simulink model "generic_IVS"  (R2024a)
settings: Solver=FixedStepDiscrete  StartTime=0.0  StopTime=inf  FixedStep=0.001  RelTol=1e-3  EnableMultiTasking=on
model workspace (MAT data in the model file):
  APPROACH = [-49.2532697283 -46.8560638421 -44.4231792578 -41.9812023919 -38.6885385845 -35.362557161 -32.0241539117 -28.6853351363 -25.3485360015 -22.0129625698 -18.6780310991 -15.3435011563 ... (76 elements, 38x2)]
  LANE_LEN = [284; 276; 267]
  LANE_XY = [59.0003214677 62.3317238784 65.6577746803 68.9711287644 72.2614514234 75.5172879138 77.9296982442 80.3117765819 82.6592727002 84.9682672017 87.2351542049 89.4565910317 ... (1704 elements, 284x2x3)]
  N_LANE = 3
  PARK_OCC = [1 1 1 1 1 1 1 1 1 1 1 1 ... (40000 elements, 200x200)]
  WB = 2.9
  branch_lane = 3
  branch_x = -49.2532697283
  branch_y = 17.3349288561
  cruise_lane = 1
  entrance_x = 6
  entrance_y = -36.6
  lane_width = 3.5
  park_goal = [21.4; -44.3; 1.57079632679]
  toll_lane = 1
  toll_post = 20
  toll_pre = 45
  toll_station = 202.6
  toll_x = -176.17
  toll_y = -85.66
  v_cruise = 11
  v_park = 2.78
  waypoints = [-81.8048181182 -79.1416974235 -76.4199514846 -73.3097017696 -70.5703457405 -67.625901331 -64.4903894371 -61.1945301864 -57.8351626085 -54.4642235015 -51.0966947204 -47.7361432477 ... (1754 elements, 877x2)]
libraries: CarMaker4SL x57, simulink x1
(part 4 of 4)

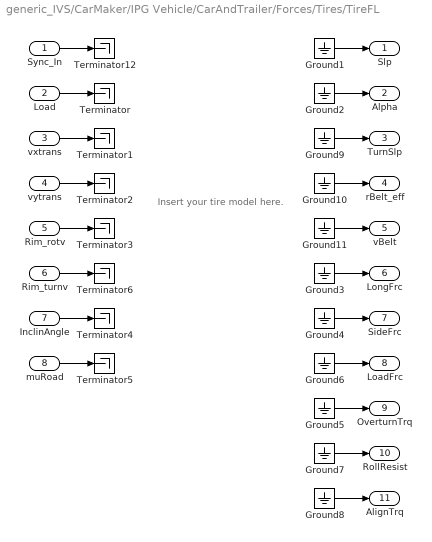
== system generic_IVS/CarMaker/IPG Vehicle/CarAndTrailer/Forces/Tires/TireFL ==
  note: Insert your tire model here.
  Sync_In : Inport
  Load : Inport  Port=2
  vxtrans : Inport  Port=3
  vytrans : Inport  Port=4
  Rim_rotv : Inport  Port=5
  Rim_turnv : Inport  Port=6
  InclinAngle : Inport  Port=7
  muRoad : Inport  Port=8
  Ground{1..11} (11 alike) : Ground
  Terminator{,1..6,12} (8 alike) : Terminator
  Slp : Outport  VectorParamsAs1DForOutWhenUnconnected=off
  Alpha : Outport  Port=2  VectorParamsAs1DForOutWhenUnconnected=off
  TurnSlp : Outport  Port=3  VectorParamsAs1DForOutWhenUnconnected=off
  rBelt_eff : Outport  Port=4  VectorParamsAs1DForOutWhenUnconnected=off
  vBelt : Outport  Port=5  VectorParamsAs1DForOutWhenUnconnected=off
  LongFrc : Outport  Port=6  VectorParamsAs1DForOutWhenUnconnected=off
  SideFrc : Outport  Port=7  VectorParamsAs1DForOutWhenUnconnected=off
  LoadFrc : Outport  Port=8  VectorParamsAs1DForOutWhenUnconnected=off
  OverturnTrq : Outport  Port=9  VectorParamsAs1DForOutWhenUnconnected=off
  RollResist : Outport  Port=10  VectorParamsAs1DForOutWhenUnconnected=off
  AlignTrq : Outport  Port=11  VectorParamsAs1DForOutWhenUnconnected=off
  wires:
  Ground11/1 -> vBelt/1
  Ground10/1 -> rBelt_eff/1
  Ground9/1 -> TurnSlp/1
  Rim_turnv/1 -> Terminator6/1
  Sync_In/1 -> Terminator12/1
  Ground2/1 -> Alpha/1
  Ground3/1 -> LongFrc/1
  Ground4/1 -> SideFrc/1
  Ground5/1 -> OverturnTrq/1
  vxtrans/1 -> Terminator1/1
  vytrans/1 -> Terminator2/1
  Rim_rotv/1 -> Terminator3/1
  InclinAngle/1 -> Terminator4/1
  muRoad/1 -> Terminator5/1
  Load/1 -> Terminator/1
  Ground1/1 -> Slp/1
  Ground6/1 -> LoadFrc/1
  Ground7/1 -> RollResist/1
  Ground8/1 -> AlignTrq/1

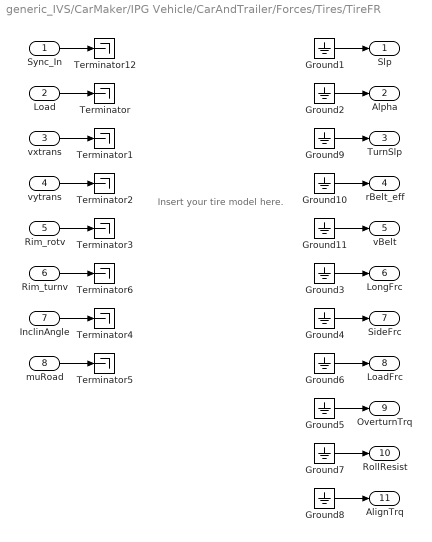
== system generic_IVS/CarMaker/IPG Vehicle/CarAndTrailer/Forces/Tires/TireFR ==
  note: Insert your tire model here.
  Sync_In : Inport
  Load : Inport  Port=2
  vxtrans : Inport  Port=3
  vytrans : Inport  Port=4
  Rim_rotv : Inport  Port=5
  Rim_turnv : Inport  Port=6
  InclinAngle : Inport  Port=7
  muRoad : Inport  Port=8
  Ground{1..11} (11 alike) : Ground
  Terminator{,1..6,12} (8 alike) : Terminator
  Slp : Outport  VectorParamsAs1DForOutWhenUnconnected=off
  Alpha : Outport  Port=2  VectorParamsAs1DForOutWhenUnconnected=off
  TurnSlp : Outport  Port=3  VectorParamsAs1DForOutWhenUnconnected=off
  rBelt_eff : Outport  Port=4  VectorParamsAs1DForOutWhenUnconnected=off
  vBelt : Outport  Port=5  VectorParamsAs1DForOutWhenUnconnected=off
  LongFrc : Outport  Port=6  VectorParamsAs1DForOutWhenUnconnected=off
  SideFrc : Outport  Port=7  VectorParamsAs1DForOutWhenUnconnected=off
  LoadFrc : Outport  Port=8  VectorParamsAs1DForOutWhenUnconnected=off
  OverturnTrq : Outport  Port=9  VectorParamsAs1DForOutWhenUnconnected=off
  RollResist : Outport  Port=10  VectorParamsAs1DForOutWhenUnconnected=off
  AlignTrq : Outport  Port=11  VectorParamsAs1DForOutWhenUnconnected=off
  wires:
  Ground11/1 -> vBelt/1
  Ground10/1 -> rBelt_eff/1
  Ground9/1 -> TurnSlp/1
  Rim_turnv/1 -> Terminator6/1
  Sync_In/1 -> Terminator12/1
  Ground2/1 -> Alpha/1
  Ground3/1 -> LongFrc/1
  Ground4/1 -> SideFrc/1
  Ground5/1 -> OverturnTrq/1
  vxtrans/1 -> Terminator1/1
  vytrans/1 -> Terminator2/1
  Rim_rotv/1 -> Terminator3/1
  InclinAngle/1 -> Terminator4/1
  muRoad/1 -> Terminator5/1
  Load/1 -> Terminator/1
  Ground1/1 -> Slp/1
  Ground6/1 -> LoadFrc/1
  Ground7/1 -> RollResist/1
  Ground8/1 -> AlignTrq/1

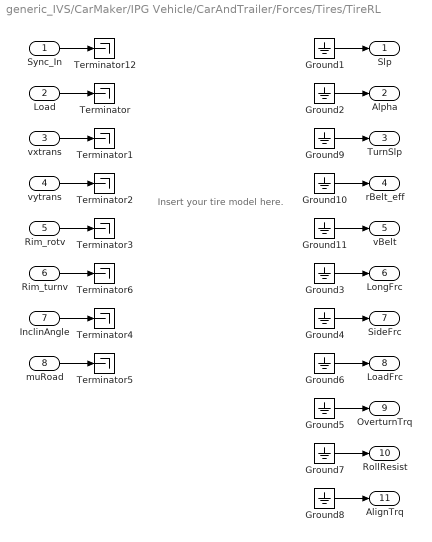
== system generic_IVS/CarMaker/IPG Vehicle/CarAndTrailer/Forces/Tires/TireRL ==
  note: Insert your tire model here.
  Sync_In : Inport
  Load : Inport  Port=2
  vxtrans : Inport  Port=3
  vytrans : Inport  Port=4
  Rim_rotv : Inport  Port=5
  Rim_turnv : Inport  Port=6
  InclinAngle : Inport  Port=7
  muRoad : Inport  Port=8
  Ground{1..11} (11 alike) : Ground
  Terminator{,1..6,12} (8 alike) : Terminator
  Slp : Outport  VectorParamsAs1DForOutWhenUnconnected=off
  Alpha : Outport  Port=2  VectorParamsAs1DForOutWhenUnconnected=off
  TurnSlp : Outport  Port=3  VectorParamsAs1DForOutWhenUnconnected=off
  rBelt_eff : Outport  Port=4  VectorParamsAs1DForOutWhenUnconnected=off
  vBelt : Outport  Port=5  VectorParamsAs1DForOutWhenUnconnected=off
  LongFrc : Outport  Port=6  VectorParamsAs1DForOutWhenUnconnected=off
  SideFrc : Outport  Port=7  VectorParamsAs1DForOutWhenUnconnected=off
  LoadFrc : Outport  Port=8  VectorParamsAs1DForOutWhenUnconnected=off
  OverturnTrq : Outport  Port=9  VectorParamsAs1DForOutWhenUnconnected=off
  RollResist : Outport  Port=10  VectorParamsAs1DForOutWhenUnconnected=off
  AlignTrq : Outport  Port=11  VectorParamsAs1DForOutWhenUnconnected=off
  wires:
  Ground11/1 -> vBelt/1
  Ground10/1 -> rBelt_eff/1
  Ground9/1 -> TurnSlp/1
  Rim_turnv/1 -> Terminator6/1
  Sync_In/1 -> Terminator12/1
  Ground2/1 -> Alpha/1
  Ground3/1 -> LongFrc/1
  Ground4/1 -> SideFrc/1
  Ground5/1 -> OverturnTrq/1
  vxtrans/1 -> Terminator1/1
  vytrans/1 -> Terminator2/1
  Rim_rotv/1 -> Terminator3/1
  InclinAngle/1 -> Terminator4/1
  muRoad/1 -> Terminator5/1
  Load/1 -> Terminator/1
  Ground1/1 -> Slp/1
  Ground6/1 -> LoadFrc/1
  Ground7/1 -> RollResist/1
  Ground8/1 -> AlignTrq/1

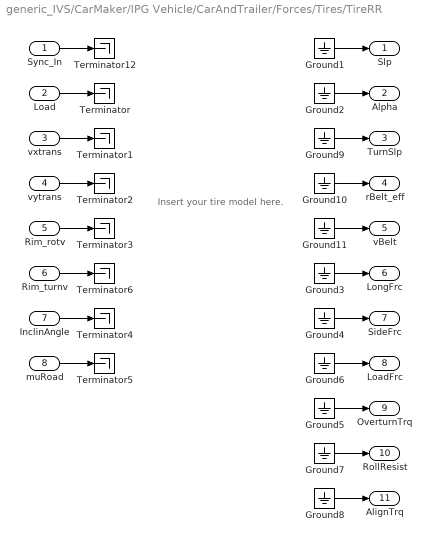
== system generic_IVS/CarMaker/IPG Vehicle/CarAndTrailer/Forces/Tires/TireRR ==
  note: Insert your tire model here.
  Sync_In : Inport
  Load : Inport  Port=2
  vxtrans : Inport  Port=3
  vytrans : Inport  Port=4
  Rim_rotv : Inport  Port=5
  Rim_turnv : Inport  Port=6
  InclinAngle : Inport  Port=7
  muRoad : Inport  Port=8
  Ground{1..11} (11 alike) : Ground
  Terminator{,1..6,12} (8 alike) : Terminator
  Slp : Outport  VectorParamsAs1DForOutWhenUnconnected=off
  Alpha : Outport  Port=2  VectorParamsAs1DForOutWhenUnconnected=off
  TurnSlp : Outport  Port=3  VectorParamsAs1DForOutWhenUnconnected=off
  rBelt_eff : Outport  Port=4  VectorParamsAs1DForOutWhenUnconnected=off
  vBelt : Outport  Port=5  VectorParamsAs1DForOutWhenUnconnected=off
  LongFrc : Outport  Port=6  VectorParamsAs1DForOutWhenUnconnected=off
  SideFrc : Outport  Port=7  VectorParamsAs1DForOutWhenUnconnected=off
  LoadFrc : Outport  Port=8  VectorParamsAs1DForOutWhenUnconnected=off
  OverturnTrq : Outport  Port=9  VectorParamsAs1DForOutWhenUnconnected=off
  RollResist : Outport  Port=10  VectorParamsAs1DForOutWhenUnconnected=off
  AlignTrq : Outport  Port=11  VectorParamsAs1DForOutWhenUnconnected=off
  wires:
  Ground11/1 -> vBelt/1
  Ground10/1 -> rBelt_eff/1
  Ground9/1 -> TurnSlp/1
  Rim_turnv/1 -> Terminator6/1
  Sync_In/1 -> Terminator12/1
  Ground2/1 -> Alpha/1
  Ground3/1 -> LongFrc/1
  Ground4/1 -> SideFrc/1
  Ground5/1 -> OverturnTrq/1
  vxtrans/1 -> Terminator1/1
  vytrans/1 -> Terminator2/1
  Rim_rotv/1 -> Terminator3/1
  InclinAngle/1 -> Terminator4/1
  muRoad/1 -> Terminator5/1
  Load/1 -> Terminator/1
  Ground1/1 -> Slp/1
  Ground6/1 -> LoadFrc/1
  Ground7/1 -> RollResist/1
  Ground8/1 -> AlignTrq/1

== matlab function generic_IVS/CarMaker/IVS_Control/LongitudinalController/lonctrl ==
  data: Traj input; ax output; Ego input
function ax = lonctrl(Traj, Ego)
%#codegen
target=Traj(3); v=Ego(4); ax=0.6*(target-v);
if ax>3; ax=3; elseif ax<-4; ax=-4; end
end

== matlab function generic_IVS/CarMaker/IVS_Control/Safety/safety ==
  data: Steer input; CFL output; Accel input; Ego input; OF input; Path input; Mode input; P_Ax input; P_Sfl input; P_Sfr input; P_Gear input; CFR output; Ax output; Gear output
function [CFL, CFR, Ax, Gear] = safety(Steer, Accel, Ego, OF, Path, Mode, P_Ax, P_Sfl, P_Sfr, P_Gear)
%#codegen
persistent prev_st; if isempty(prev_st); prev_st=0; end
ev=Ego(4); tx=Ego(1); ty=Ego(2); ua=Mode(4);
Np=numel(Path)/2; No=floor(numel(OF)/8); slen=zeros(Np,1); px=tx;py=ty;
for j=1:Np; qx=Path(2*j-1);qy=Path(2*j); seg=sqrt((qx-px)^2+(qy-py)^2); if j==1; slen(j)=seg; else; slen(j)=slen(j-1)+seg; end; px=qx;py=qy; end
emerg=false;
for i=1:No
  o=(i-1)*8; if OF(o+8)<0.5; continue; end
  ox=OF(o+1); oy=OF(o+2); xr=OF(o+3); yr=OF(o+4); vrel=OF(o+5); vyr=OF(o+6); dist=OF(o+7);
  if ua>0.5
    if dist<0.8; emerg=true; end
  else
    if dist<1.4 && ev>5; emerg=true; end
    if ev>5 && dist<5.5 && abs(xr)<7 && abs(yr)<4 && yr*vyr<-0.4; emerg=true; end
    dmin=inf; jm=1; for j=1:Np; dx=Path(2*j-1)-ox; dy=Path(2*j)-oy; d=dx*dx+dy*dy; if d<dmin; dmin=d; jm=j; end; end
    dcross=sqrt(dmin); s=slen(jm);
    if dcross<1.8 && s>0.3 && s<25; ttc=inf; if vrel<-0.2; ttc=s/(-vrel); end; if ttc<1.0 || s<3.5; emerg=true; end; end
  end
end
ax=Accel; if emerg; ax=-4.0; end; if ax>3; ax=3; elseif ax<-4; ax=-4; end
st=prev_st+0.12*(Steer-prev_st); if st>0.5; st=0.5; elseif st<-0.5; st=-0.5; end; prev_st=st;
if Mode(5)>0.5
  CFL=P_Sfl; CFR=P_Sfr; Ax=P_Ax; Gear=P_Gear;
else
  CFL=st; CFR=st; Ax=ax; Gear=1.0;
end
end

== matlab function generic_IVS/CarMaker/IVS_Control/ObjectManager/objmgr ==
  data: Obs input; ObsFeat output; Ego input
function ObsFeat = objmgr(Obs, Ego)
%#codegen
ex=Ego(1); ey=Ego(2); erz=Ego(3); ev=Ego(4); c=cos(erz); s=sin(erz);
ObsFeat=zeros(232,1);
for i=1:29
  if i<=16; b=(i-1)*5; gx=Obs(b+1); gy=Obs(b+2); vgx=0; vgy=0;
  else; b=80+(i-17)*10; gx=Obs(b+1); gy=Obs(b+2); vgx=Obs(b+4); vgy=Obs(b+5); end
  dx=gx-ex; dy=gy-ey; xr=c*dx+s*dy; yr=-s*dx+c*dy;
  vxr=c*vgx+s*vgy-ev; vyr=-s*vgx+c*vgy; dist=sqrt(dx*dx+dy*dy);
  vv=0; if (abs(gx)>0.1||abs(gy)>0.1) && dist<200; vv=1; end
  o=(i-1)*8; ObsFeat(o+1)=gx; ObsFeat(o+2)=gy; ObsFeat(o+3)=xr; ObsFeat(o+4)=yr; ObsFeat(o+5)=vxr; ObsFeat(o+6)=vyr; ObsFeat(o+7)=dist; ObsFeat(o+8)=vv;
end
end

== matlab function generic_IVS/CarMaker/IVS_Control/Parking/parking_wrap ==
  data: Ego input; ax output; Mode input; goal input; occ input; sfl output; sfr output; gear output
function [ax,sfl,sfr,gear] = parking_wrap(Ego, Mode, goal, occ)
%#codegen
persistent armed; if isempty(armed); armed=false; end
if Mode(5)>0.5; armed=true; end
if armed
  [ax,sfl,sfr,gear]=pp_parking(Ego(1),Ego(2),Ego(3),Ego(4),[0;0],[goal(1);goal(2)],goal(3),occ);
else
  ax=0.0; sfl=0.0; sfr=0.0; gear=-9.0;
end
end

== stateflow chart generic_IVS/CarMaker/Subsystem/Day3/Chart ==
  (default) -> (junction 1)
  (junction 1) -> (junction 3) [order 1] : [i<99]
      | {i = i + 1;}
  (junction 1) -> (junction 7) [order 2] : {i=0;}
  (junction 3) -> (junction 5)
  (junction 5) -> (junction 7)
  (junction 7) -> (junction 10)
  (junction 10) -> (junction 12) [order 1] : [rem(i,50) == 0]
      | {do_Logic;}
  (junction 10) -> (junction 18) [order 2]
  (junction 12) -> (junction 16)
  (junction 16) -> (junction 18)
  (junction 18) -> (junction 21)
  data: i local =0
  events: do_Logic output FUNCTION_CALL_EVENT

== stateflow chart generic_IVS/CarMaker/IVS_Control/Chart ==
  settings: updateMethod=DISCRETE  sampleTime=0.001
  (default) -> (junction 1)
  (junction 1) -> (junction 3) [order 1] : [mod(i,10) == 0]
      | {do_Logic_10ms;}
  (junction 1) -> (junction 7) [order 2]
  (junction 3) -> (junction 5)
  (junction 5) -> (junction 7)
  (junction 7) -> (junction 10)
  (junction 10) -> (junction 12) [order 1] : [mod(i, 50) == 0]
      | {do_Logic_50ms;}
  (junction 10) -> (junction 18) [order 2]
  (junction 12) -> (junction 16)
  (junction 16) -> (junction 18)
  (junction 18) -> (junction 25)
  (junction 25) -> (junction 27) [order 1] : [mod(i,100) == 0]
      | {do_Logic_100ms;}
  (junction 25) -> (junction 21) [order 2]
  (junction 27) -> (junction 29) : {i = 0;}
  (junction 29) -> (junction 21)
  (junction 21) -> (junction 32) : {i = i +1;}
  data: i local =0
  events: do_Logic_10ms output FUNCTION_CALL_EVENT; do_Logic_50ms output FUNCTION_CALL_EVENT; do_Logic_100ms output FUNCTION_CALL_EVENT

== matlab function generic_IVS/CarMaker/IVS_Control/ModeManager/modemgr ==
  data: Ego input; Mode output; OF input; LANE_XY input; LANE_LEN input; cruise_lane input; v_cruise input; v_park input; lane_width input; branch_lane input; toll_lane input; toll_x input; toll_y input; branch_x input; branch_y input; entrance_x input; entrance_y input
function Mode = modemgr(Ego, OF, LANE_XY, LANE_LEN, cruise_lane, v_cruise, v_park, lane_width, branch_lane, toll_lane, toll_x, toll_y, branch_x, branch_y, entrance_x, entrance_y)
%#codegen
persistent committed toll_reached toll_done go_park on_appr lc_cool ph bypass astk
if isempty(committed); committed=double(cruise_lane); toll_reached=false; toll_done=false; go_park=false; on_appr=false; lc_cool=0; ph=Ego(3); bypass=false; astk=0; end
tx=Ego(1); ty=Ego(2); ev=Ego(4); nL=size(LANE_XY,3); No=floor(numel(OF)/8);
if lc_cool>0; lc_cool=lc_cool-1; end
dh=Ego(3)-ph; if dh>pi; dh=dh-2*pi; elseif dh<-pi; dh=dh+2*pi; end; ph=Ego(3); yawing=abs(dh)>0.004;
fwd=inf(nL,1); blocked=false(nL,1);
for i=1:No
  o=(i-1)*8; if OF(o+8)<0.5; continue; end
  ox=OF(o+1); oy=OF(o+2); xr=OF(o+3);
  bl=1; bd=inf;
  for li=1:nL
    n=LANE_LEN(li); dm=inf;
    for k=1:n; dx=LANE_XY(k,1,li)-ox; dy=LANE_XY(k,2,li)-oy; d=dx*dx+dy*dy; if d<dm; dm=d; end; end
    if dm<bd; bd=dm; bl=li; end
  end
  if sqrt(bd)>lane_width*0.6; continue; end
  if xr>0.5 && xr<fwd(bl); fwd(bl)=xr; end
  if xr>-13 && xr<22; blocked(bl)=true; end
end
cr=double(cruise_lane); dtoll=sqrt((tx-toll_x)^2+(ty-toll_y)^2); dbr=sqrt((tx-branch_x)^2+(ty-branch_y)^2);
if ~toll_done; if dtoll<8; toll_reached=true; end; if toll_reached && dtoll>15; toll_done=true; go_park=true; end; end
toll_lock = ~toll_done && dtoll<25;
if go_park && ~bypass && dbr<35 && ev<0.4; astk=astk+1; else; astk=0; end
if astk>160; bypass=true; on_appr=false; astk=0; committed=cr; end
if bypass && dbr>70; bypass=false; end
ovtk_ok = ~toll_lock && ~on_appr && lc_cool==0 && ~yawing && (~go_park || dbr>60 || bypass);
if ovtk_ok
  cl=committed;
  if fwd(cl)<35
    bestc=cl; bestg=fwd(cl);
    for dlt=[-1 1]
      cand=cl+dlt;
      if cand>=1 && cand<=nL && ~blocked(cand) && fwd(cand)>bestg+8; bestc=cand; bestg=fwd(cand); end
    end
    if bestc~=committed; committed=bestc; lc_cool=50; end
  elseif committed~=cr && ~blocked(cr) && fwd(cr)>40
    committed=cr; lc_cool=50;
  end
end
tl=committed; vset=v_cruise; stop=0; use_appr=0; pr=0;
if toll_lock; tl=double(toll_lane); committed=double(toll_lane); end
if go_park && ~bypass
  if on_appr || dbr<20
    on_appr=true; use_appr=1; vset=v_park; tl=double(branch_lane); committed=double(branch_lane);
  elseif dbr<40
    tl=double(branch_lane); committed=double(branch_lane); vset=8;
  elseif dbr<60
    tl=2; if nL>=2; committed=2; end; vset=10;
  else
    vset=10;
  end
  dent=sqrt((tx-entrance_x)^2+(ty-entrance_y)^2);
  if on_appr && dent<4.0; stop=1; if ev<0.3; pr=1; end; end
end
Mode=[tl; vset; stop; use_appr; pr];
end

== matlab function generic_IVS/CarMaker/IVS_Control/MapManager/mapmgr ==
  data: Ego input; MapCtx output; LANE_XY input; LANE_LEN input
function MapCtx = mapmgr(Ego, LANE_XY, LANE_LEN)
%#codegen
tx=Ego(1); ty=Ego(2); nL=size(LANE_XY,3);
cur=1; bestd=inf; sidx=1;
for li=1:nL
  n=LANE_LEN(li); dmin=inf; im=1;
  for k=1:n
    dx=LANE_XY(k,1,li)-tx; dy=LANE_XY(k,2,li)-ty; d=dx*dx+dy*dy;
    if d<dmin; dmin=d; im=k; end
  end
  if dmin<bestd; bestd=dmin; cur=li; sidx=im; end
end
MapCtx=[cur; sidx; sidx/max(1,LANE_LEN(cur)); sqrt(bestd)];
end

== matlab function generic_IVS/CarMaker/IVS_Control/PathPlanning/pathplan ==
  data: Ego input; Path output; Mode input; LANE_XY input; LANE_LEN input; APPROACH input
function Path = pathplan(Ego, Mode, LANE_XY, LANE_LEN, APPROACH)
%#codegen
Np=30; tx=Ego(1); ty=Ego(2); Path=zeros(2*Np,1);
if Mode(4)>0.5
  n=size(APPROACH,1); dmin=inf; im=1;
  for k=1:n; dx=APPROACH(k,1)-tx; dy=APPROACH(k,2)-ty; d=dx*dx+dy*dy; if d<dmin; dmin=d; im=k; end; end
  for j=1:Np; idx=im+(j-1); if idx>n; idx=n; end; Path(2*j-1)=APPROACH(idx,1); Path(2*j)=APPROACH(idx,2); end
else
  nL=size(LANE_XY,3); tl=round(Mode(1)); if tl<1; tl=1; elseif tl>nL; tl=nL; end
  n=LANE_LEN(tl); dmin=inf; im=1;
  for k=1:n; dx=LANE_XY(k,1,tl)-tx; dy=LANE_XY(k,2,tl)-ty; d=dx*dx+dy*dy; if d<dmin; dmin=d; im=k; end; end
  for j=1:Np; idx=mod(im-1+(j-1), n)+1; Path(2*j-1)=LANE_XY(idx,1,tl); Path(2*j)=LANE_XY(idx,2,tl); end
end
end

== matlab function generic_IVS/CarMaker/IVS_Control/TrajectoryPlanning/trajplan ==
  data: Path input; Traj output; Ego input; Mode input; OF input
function Traj = trajplan(Path, Ego, Mode, OF)
%#codegen
Np=numel(Path)/2; v=Ego(4); tx=Ego(1); ty=Ego(2);
Ld=6+0.6*v; if Ld<11; Ld=11; elseif Ld>18; Ld=18; end
px=tx;py=ty;accL=0;lax=Path(1);lay=Path(2); slen=zeros(Np,1);
for j=1:Np; qx=Path(2*j-1);qy=Path(2*j); seg=sqrt((qx-px)^2+(qy-py)^2); if j==1; slen(j)=seg; else; slen(j)=slen(j-1)+seg; end; accL=accL+seg; if accL<=Ld; lax=qx; lay=qy; end; px=qx;py=qy; end
ts=Mode(2); sf=Mode(3); ua=Mode(4); if sf>0.5; ts=0; end
if ua<0.5
  No=floor(numel(OF)/8); lead_s=inf; lead_vrel=0;
  for i=1:No
    o=(i-1)*8; if OF(o+8)<0.5; continue; end
    ox=OF(o+1); oy=OF(o+2); dmin=inf; jm=1;
    for j=1:Np; dx=Path(2*j-1)-ox; dy=Path(2*j)-oy; d=dx*dx+dy*dy; if d<dmin; dmin=d; jm=j; end; end
    if sqrt(dmin)<1.6 && slen(jm)>1 && slen(jm)<55 && slen(jm)<lead_s; lead_s=slen(jm); lead_vrel=OF(o+5); end
  end
  if isfinite(lead_s); des=6+1.2*v; va=v+lead_vrel+0.45*(lead_s-des); if va<0; va=0; end; if va<ts; ts=va; end; end
end
Traj=[lax; lay; ts; sf];
end

== matlab function generic_IVS/CarMaker/IVS_Control/LateralController/latctrl ==
  data: Traj input; steer output; Ego input; WB input
function steer = latctrl(Traj, Ego, WB)
%#codegen
tx=Ego(1); ty=Ego(2); rz=Ego(3); lax=Traj(1); lay=Traj(2);
c=cos(rz); s=sin(rz); ex=lax-tx; ey=lay-ty;
xv=c*ex+s*ey; yv=-s*ex+c*ey; Ld=sqrt(xv*xv+yv*yv); if Ld<1e-3; Ld=1e-3; end
alpha=atan2(yv,xv); delta=atan2(2*WB*sin(alpha),Ld);
if delta>0.5; delta=0.5; elseif delta<-0.5; delta=-0.5; end
steer=delta;
end
